simulink model "pulse_detector_axis_zcu111_fil_interface"  (R2019b)
settings: Solver=FixedStepDiscrete  StartTime=0.0  StopTime=1  FixedStep=1  RelTol=1e-3  EnableMultiTasking=on
PreLoadFcn:
  | model_init
  | load FIL_axis_data_in
InitFcn:
  | model_init;
  | load FIL_axis_data_in
  | matlabshared.libiio.internal.ContextManager.reset
undefined symbols (not defined in the file or in its folder): FIL_axis_data_in
libraries: hdlsllib x3, psp_axi_iio_lib x2
settings Model: LastModifiedBy=ajtro
settings SolverCC: PositivePriorityOrder=on
settings DataIOCC: SaveOutput=off  SaveTime=off  ReturnWorkspaceOutputs=off
settings OptimizationCC: BlockReduction=off  ConditionallyExecuteInputs=off  EnhancedBackFolding=on  PassReuseOutputArgsAs=Individual arguments  MaxStackSize=64  OptimizeBlockOrder=speed  DifferentSizesBufferReuse=on  OptimizationCustomize=off  EfficientTunableParamExpr=on
settings DebuggingCC: AlgebraicLoopMsg=error  SingleTaskRateTransMsg=error  ParameterTunabilityLossMsg=error  PregeneratedLibrarySubsystemCodeDiagnostic=none  StrictBusMsg=ErrorOnBusTreatedAsVector  SFUnexpectedBacktrackingDiag=warning  SFNoUnconditionalDefaultTransitionDiag=warning  SFExecutionAtInitializationDiag=none  ArithmeticOperatorsInVariantConditions=warning
settings HardwareCC: ProdBitPerLong=64  ProdLargestAtomicInteger=LongLong  ProdLargestAtomicFloat=Double  ProdLongLongMode=on  ProdHWDeviceType=ARM Compatible->ARMv8 Cortex-A (AArch64)  TargetBitPerLong=64  TargetBitPerPointer=64  TargetBitPerSizeT=64  TargetBitPerPtrDiffT=64  TargetLargestAtomicInteger=LongLong  TargetLargestAtomicFloat=Double  TargetLongLongMode=on  TargetIntDivRoundTo=Zero  TargetEndianess=LittleEndian  TargetWordSize=64  TargetHWDeviceType=ARM Compatible->ARM 64-bit (LP64)
settings SFSimCC: SimUseLocalCustomCode=off  MATLABDynamicMemAlloc=off  CustomCodeUndefinedFunction=UseInterfaceOnly
settings RTWCC: SystemTargetFile=ert.tlc  HardwareBoard=Xilinx Zynq Ultrascale RFSoC based board  TLCOptions="-aInlineSetEventsForThisBaseRateFcn=TLC_FALSE -aSuppressMultiTaskScheduler=TLC_FALSE  -aRateBasedStepFcn=0"  TemplateMakefile=ert_default_tmf  GenerateReport=on  RTWUseLocalCustomCode=off  Toolchain=Linaro AArch64 Linux Toolchain Toolchain v6.3  IncludeHyperlinkInReport=on  LaunchReport=on  GenerateTraceInfo=on  GenerateTraceReport=on  GenerateTraceReportSl=on  GenerateTraceReportSf=on  GenerateTraceReportEml=on
settings CodeAppCC: ForceParamTrailComments=on  IgnoreCustomStorageClasses=off  OperatorAnnotations=on  SimulinkDataObjDesc=on  SFDataObjDesc=on  InsertBlockDesc=on
settings ConfigComp: CovMetricSettings=dw  CovHtmlReporting=on  CovSaveCumulativeToWorkspaceVar=on  CovSaveSingleToWorkspaceVar=on  CovExternalEMLEnable=off

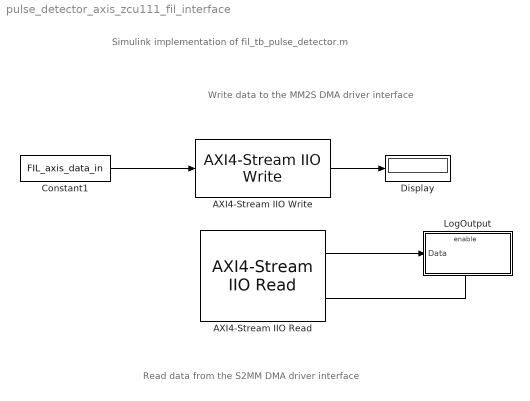
== system pulse_detector_axis_zcu111_fil_interface ==
  note: Simulink implementation of fil_tb_pulse_detector.m
  note: Read data from the S2MM DMA driver interface
  note: Write data to the MM2S DMA driver interface
  " LogOutput" : Subsystem
  AXI4-Stream IIO Read : psp_axi_iio_lib/AXI4-Stream IIO Read  SamplesPerFrame=length(FIL_axis_data_in)  DataType=ufix128  Timeout=0.1  IPAddress=192.168.1.101  enIO=on  devName=mwipcore0:s2mm0  IPResetMode=none  TLASTMode=auto  TLASTResetMode=prebuffer
      settings: SourceProductName=IIO AXI - PSP
  AXI4-Stream IIO Write : psp_axi_iio_lib/AXI4-Stream IIO Write  Timeout=0.1  IPAddress=192.168.1.101  enIO=on  devName=mwipcore0:mm2s0  IPResetMode=none
      settings: SourceProductName=IIO AXI - PSP
  Constant1 : Constant  Value=FIL_axis_data_in  SampleTime=-1
  Display : Display
  wires:
  AXI4-Stream IIO Write/1 -> Display/1
  AXI4-Stream IIO Read/1 -> " LogOutput"/1(Data)
  AXI4-Stream IIO Read/2 -> " LogOutput"/Enable
  Constant1/1 -> AXI4-Stream IIO Write/1

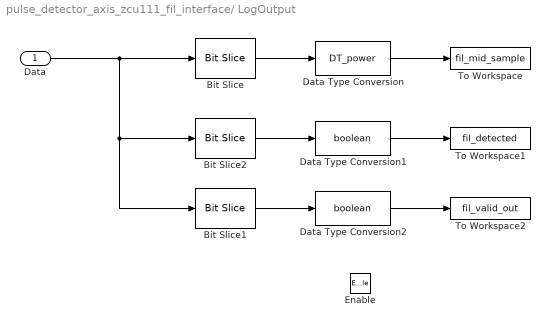
== system pulse_detector_axis_zcu111_fil_interface/ LogOutput ==
  Data : Inport
  Enable : EnablePort
  Bit Slice : hdlsllib/Logic and Bit Operations/Bit Slice  lidx=19  ridx=2
      settings: SourceProductName=Simulink  SourceProductBaseCode=SL
  Bit Slice1 : hdlsllib/Logic and Bit Operations/Bit Slice  lidx=0  ridx=0
      settings: SourceProductName=Simulink  SourceProductBaseCode=SL
  Bit Slice2 : hdlsllib/Logic and Bit Operations/Bit Slice  lidx=1  ridx=1
      settings: SourceProductName=Simulink  SourceProductBaseCode=SL
  Data Type Conversion : DataTypeConversion  OutDataTypeStr=DT_power  ConvertRealWorld=Stored Integer (SI)
  Data Type Conversion1 : DataTypeConversion  OutDataTypeStr=boolean
  Data Type Conversion2 : DataTypeConversion  OutDataTypeStr=boolean
  To Workspace : ToWorkspace  VariableName=fil_mid_sample  SampleTime=-1
      settings: Save2DSignal=2-D array (concatenate along first dimension)
  To Workspace1 : ToWorkspace  VariableName=fil_detected  SampleTime=-1
      settings: Save2DSignal=2-D array (concatenate along first dimension)
  To Workspace2 : ToWorkspace  VariableName=fil_valid_out  SampleTime=-1
      settings: Save2DSignal=2-D array (concatenate along first dimension)
  wires:
  Bit Slice1/1 -> Data Type Conversion2/1
  Data Type Conversion2/1 -> To Workspace2/1
  Data Type Conversion1/1 -> To Workspace1/1
  Bit Slice2/1 -> Data Type Conversion1/1
  Data Type Conversion/1 -> To Workspace/1
  Bit Slice/1 -> Data Type Conversion/1
  Data/1 -> Bit Slice/1, Bit Slice2/1, Bit Slice1/1
